simulink model "pod_traverse_model"  (R2021b)
settings: Solver=VariableStepAuto  StartTime=0.0  StopTime=10.0  RelTol=1e-3
settings Model: Creator=noait  LastModifiedBy=noait

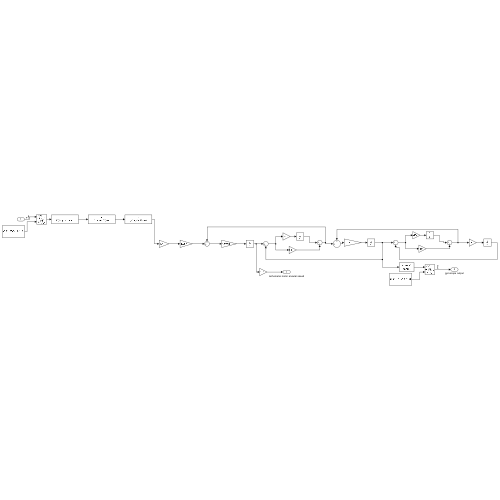
[thumbnail: Simulink's stored preview of the top-level diagram]
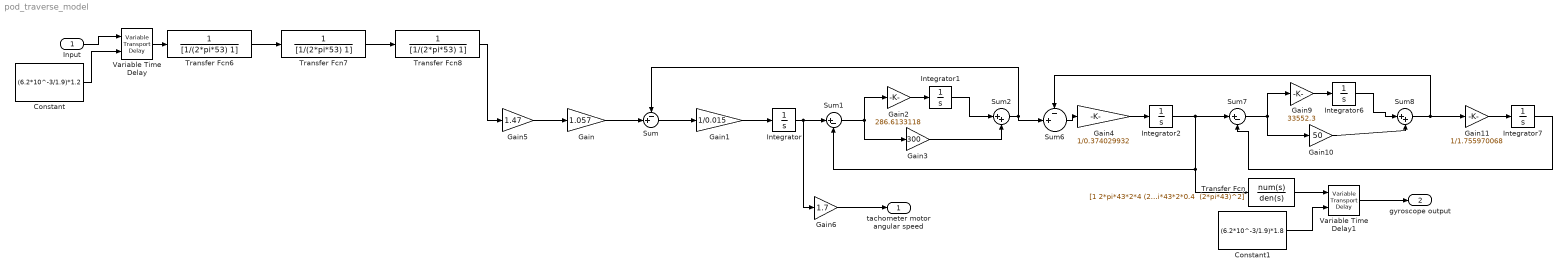
== system pod_traverse_model ==
  Input : Inport
  Constant : Constant  Value=(6.2*10^-3/1.9)*1.2  SampleTime=-1
  Constant1 : Constant  Value=(6.2*10^-3/1.9)*1.8  SampleTime=-1
  Gain : Gain  Gain=1.057
  Gain1 : Gain  Gain=1/0.015
  Gain10 : Gain  Gain=50
  Gain11 : Gain  Gain=1/1.755970068
  Gain2 : Gain  Gain=286.6133118
  Gain3 : Gain  Gain=300
  Gain4 : Gain  Gain=1/0.374029932
  Gain5 : Gain  Gain=1.47
  Gain6 : Gain  Gain=1.7
  Gain9 : Gain  Gain=33552.3
  Integrator{,1..2,6..7} (5 alike) : Integrator
  Sum : Sum  Inputs=-+|
  Sum1 : Sum  Inputs=|+-
  Sum2 : Sum  Inputs=|++
  Sum6 : Sum  Inputs=-+|
  Sum7 : Sum  Inputs=|+-
  Sum8 : Sum  Inputs=|++
  Transfer Fcn : TransferFcn  Numerator=[1 2*pi*43*2*4 (2*pi*43)^2]  Denominator="[1 2*pi*43*2*0.4  (2*pi*43)^2]"
  Transfer Fcn6 : TransferFcn  Denominator=[1/(2*pi*53) 1]
  Transfer Fcn7 : TransferFcn  Denominator=[1/(2*pi*53) 1]
  Transfer Fcn8 : TransferFcn  Denominator=[1/(2*pi*53) 1]
  Variable Time Delay : VariableTransportDelay  MaximumDelay=10  TransDelayFeedthrough=on
  Variable Time Delay1 : VariableTransportDelay  MaximumDelay=10  TransDelayFeedthrough=on
  tachometer motor angular speed : Outport
  gyroscope output : Outport  Port=2
  wires:
  Gain/1 -> Sum/2
  Sum/1 -> Gain1/1
  Gain1/1 -> Integrator/1
  Integrator/1 -> Gain6/1, Sum1/1
  Gain2/1 -> Integrator1/1
  Integrator1/1 -> Sum2/1
  Gain3/1 -> Sum2/2
  Sum1/1 -> Gain3/1, Gain2/1
  Sum2/1 -> Sum6/2, Sum/1
  Gain4/1 -> Integrator2/1
  Sum6/1 -> Gain4/1
  Integrator6/1 -> Sum8/1
  Gain10/1 -> Sum8/2
  Gain9/1 -> Integrator6/1
  Sum7/1 -> Gain10/1, Gain9/1
  Sum8/1 -> Gain11/1, Sum6/1
  Integrator7/1 -> Sum7/2
  Gain11/1 -> Integrator7/1
  Gain5/1 -> Gain/1
  Gain6/1 -> tachometer motor angular speed/1
  Integrator2/1 -> Sum7/1, Transfer Fcn/1, Sum1/2
  Transfer Fcn7/1 -> Transfer Fcn8/1
  Transfer Fcn6/1 -> Transfer Fcn7/1
  Transfer Fcn8/1 -> Gain5/1
  Variable Time Delay/1 -> Transfer Fcn6/1
  Input/1 -> Variable Time Delay/1
  Constant/1 -> Variable Time Delay/2
  Transfer Fcn/1 -> Variable Time Delay1/1
  Constant1/1 -> Variable Time Delay1/2
  Variable Time Delay1/1 -> gyroscope output/1
